simulink model "ATRIAS_vnmc"  (R2015a)
(part 22 of 23)

    (2*I^2*ddx_des*lambda1*lambda2*m*mu_s + L1^2*ddy_des*lambda2*lambda3*m^3*sin(gamma1)^2 + L1^2*g*lambda2*lambda3*m^3*sin(gamma1)^2 + 2*I^2*ddy_des*lambda1*lambda2*m*mu_s^2 + 2*I^2*g*lambda1*lambda2*m*mu_s^2 + L1^2*ddx_des*lambda1*lambda3*m^3*mu_s^3*cos(gamma1)^2 + L1^2*ddy_des*lambda2*lambda3*m^3*mu_s^2*cos(gamma1)^2 + L1^2*g*lambda2*lambda3*m^3*mu_s^2*cos(gamma1)^2 + 2*d^2*ddy_des*lambda2*lambda3*m^3*mu_s^2*cos(theta)^2 + 2*d^2*g*lambda2*lambda3*m^3*mu_s^2*cos(theta)^2 + L1^2*ddx_des*lambda1*lambda3*m^3*mu_s*sin(gamma1)^2 + I*L1*ddtheta_des*lambda2*lambda3*m^2*sin(gamma1) - I*L2*ddtheta_des*lambda2*lambda3*m^2*sin(gamma2) + 2*d^2*ddx_des*lambda1*lambda3*m^3*mu_s*sin(theta)^2 + 2*L1^2*ddy_des*lambda2*lambda3*m^3*mu_s*cos(gamma1)*sin(gamma1) + 2*L1^2*g*lambda2*lambda3*m^3*mu_s*cos(gamma1)*sin(gamma1) + I*L1*ddtheta_des*lambda2*lambda3*m^2*mu_s*cos(gamma1) + I*L2*ddtheta_des*lambda2*lambda3*m^2*mu_s*cos(gamma2) + 2*d^2*ddy_des*lambda2*lambda3*m^3*mu_s*cos(theta)*sin(theta) - 2*I*d*ddtheta_des*lambda2*lambda3*m^2*mu_s*cos(theta) + 2*d^2*g*lambda2*lambda3*m^3*mu_s*cos(theta)*sin(theta) + 2*L1^2*ddx_des*lambda1*lambda3*m^3*mu_s^2*cos(gamma1)*sin(gamma1) - I*L1*ddtheta_des*lambda1*lambda3*m^2*mu_s^3*cos(gamma1) + I*L2*ddtheta_des*lambda1*lambda3*m^2*mu_s^3*cos(gamma2) - I*L1*ddtheta_des*lambda1*lambda3*m^2*mu_s^2*sin(gamma1) - I*L2*ddtheta_des*lambda1*lambda3*m^2*mu_s^2*sin(gamma2) - L1*L2*ddy_des*lambda2*lambda3*m^3*sin(gamma1)*sin(gamma2) + 2*d^2*ddx_des*lambda1*lambda3*m^3*mu_s^2*cos(theta)*sin(theta) - L1*L2*g*lambda2*lambda3*m^3*sin(gamma1)*sin(gamma2) + 2*I*d*ddtheta_des*lambda1*lambda3*m^2*mu_s^2*sin(theta) - L1*d*ddy_des*lambda2*lambda3*m^3*sin(gamma1)*sin(theta) + L2*d*ddy_des*lambda2*lambda3*m^3*sin(gamma2)*sin(theta) - L1*d*g*lambda2*lambda3*m^3*sin(gamma1)*sin(theta) + L2*d*g*lambda2*lambda3*m^3*sin(gamma2)*sin(theta) - L1*L2*ddy_des*lambda2*lambda3*m^3*mu_s*cos(gamma1)*sin(gamma2) + L1*L2*ddy_des*lambda2*lambda3*m^3*mu_s*cos(gamma2)*sin(gamma1) - L1*L2*g*lambda2*lambda3*m^3*mu_s*cos(gamma1)*sin(gamma2) + L1*L2*g*lambda2*lambda3*m^3*mu_s*cos(gamma2)*sin(gamma1) + L1*L2*ddx_des*lambda1*lambda3*m^3*mu_s*sin(gamma1)*sin(gamma2) - L1*d*ddy_des*lambda2*lambda3*m^3*mu_s*cos(gamma1)*sin(theta) - 3*L1*d*ddy_des*lambda2*lambda3*m^3*mu_s*cos(theta)*sin(gamma1) - L2*d*ddy_des*lambda2*lambda3*m^3*mu_s*cos(gamma2)*sin(theta) + L2*d*ddy_des*lambda2*lambda3*m^3*mu_s*cos(theta)*sin(gamma2) - L1*d*g*lambda2*lambda3*m^3*mu_s*cos(gamma1)*sin(theta) - 3*L1*d*g*lambda2*lambda3*m^3*mu_s*cos(theta)*sin(gamma1) - L2*d*g*lambda2*lambda3*m^3*mu_s*cos(gamma2)*sin(theta) + L2*d*g*lambda2*lambda3*m^3*mu_s*cos(theta)*sin(gamma2) - 3*L1*d*ddx_des*lambda1*lambda3*m^3*mu_s*sin(gamma1)*sin(theta) - L2*d*ddx_des*lambda1*lambda3*m^3*mu_s*sin(gamma2)*sin(theta) - L1*L2*ddx_des*lambda1*lambda3*m^3*mu_s^3*cos(gamma1)*cos(gamma2) + L1*L2*ddy_des*lambda2*lambda3*m^3*mu_s^2*cos(gamma1)*cos(gamma2) + L1*L2*g*lambda2*lambda3*m^3*mu_s^2*cos(gamma1)*cos(gamma2) + L1*L2*ddx_des*lambda1*lambda3*m^3*mu_s^2*cos(gamma1)*sin(gamma2) - L1*L2*ddx_des*lambda1*lambda3*m^3*mu_s^2*cos(gamma2)*sin(gamma1) - L1*d*ddx_des*lambda1*lambda3*m^3*mu_s^3*cos(gamma1)*cos(theta) + L2*d*ddx_des*lambda1*lambda3*m^3*mu_s^3*cos(gamma2)*cos(theta) - 3*L1*d*ddy_des*lambda2*lambda3*m^3*mu_s^2*cos(gamma1)*cos(theta) - L2*d*ddy_des*lambda2*lambda3*m^3*mu_s^2*cos(gamma2)*cos(theta) - 3*L1*d*g*lambda2*lambda3*m^3*mu_s^2*cos(gamma1)*cos(theta) - L2*d*g*lambda2*lambda3*m^3*mu_s^2*cos(gamma2)*cos(theta) - 3*L1*d*ddx_des*lambda1*lambda3*m^3*mu_s^2*cos(gamma1)*sin(theta) - L1*d*ddx_des*lambda1*lambda3*m^3*mu_s^2*cos(theta)*sin(gamma1) + L2*d*ddx_des*lambda1*lambda3*m^3*mu_s^2*cos(gamma2)*sin(theta) - L2*d*ddx_des*lambda1*lambda3*m^3*mu_s^2*cos(theta)*sin(gamma2))/(4*I^2*lambda1*lambda2*mu_s^2 + L1^2*lambda2*lambda3*m^2*sin(gamma1)^2 + L2^2*lambda2*lambda3*m^2*sin(gamma2)^2 + L1^2*lambda2*lambda3*m^2*mu_s^2*cos(gamma1)^2 + L1^2*lambda1*lambda3*m^2*mu_s^4*cos(gamma1)^2 + L2^2*lambda2*lambda3*m^2*mu_s^2*cos(gamma2)^2 + L2^2*lambda1*lambda3*m^2*mu_s^4*cos(gamma2)^2 + L1^2*lambda1*lambda3*m^2*mu_s^2*sin(gamma1)^2 + L2^2*lambda1*lambda3*m^2*mu_s^2*sin(gamma2)^2 + 4*d^2*lambda2*lambda3*m^2*mu_s^2*cos(theta)^2 + 4*d^2*lambda1*lambda3*m^2*mu_s^2*sin(theta)^2 + 2*L1^2*lambda1*lambda3*m^2*mu_s^3*cos(gamma1)*sin(gamma1) - 2*L2^2*lambda1*lambda3*m^2*mu_s^3*cos(gamma2)*sin(gamma2) - 2*L1*L2*lambda2*lambda3*m^2*sin(gamma1)*sin(gamma2) + 2*L1^2*lambda2*lambda3*m^2*mu_s*cos(gamma1)*sin(gamma1) - 2*L2^2*lambda2*lambda3*m^2*mu_s*cos(gamma2)*sin(gamma2) + 2*L1*L2*lambda1*lambda3*m^2*mu_s^3*cos(gamma1)*sin(gamma2) - 2*L1*L2*lambda1*lambda3*m^2*mu_s^3*cos(gamma2)*sin(gamma1) + 2*L1*L2*lambda1*lambda3*m^2*mu_s^2*sin(gamma1)*sin(gamma2) - 4*L1*d*lambda2*lambda3*m^2*mu_s^2*cos(gamma1)*cos(theta) - 4*L2*d*lambda2*lambda3*m^2*mu_s^2*cos(gamma2)*cos(theta) - 4*L1*d*lambda1*lambda3*m^2*mu_s^3*cos(gamma1)*sin(theta) + 4*L2*d*lambda1*lambda3*m^2*mu_s^3*cos(gamma2)*sin(theta) - 4*L1*d*lambda1*lambda3*m^2*mu_s^2*sin(gamma1)*sin(theta) - 4*L2*d*lambda1*lambda3*m^2*mu_s^2*sin(gamma2)*sin(theta) - 2*L1*L2*lambda2*lambda3*m^2*mu_s*cos(gamma1)*sin(gamma2) + 2*L1*L2*lambda2*lambda3*m^2*mu_s*cos(gamma2)*sin(gamma1) - 4*L1*d*lambda2*lambda3*m^2*mu_s*cos(theta)*sin(gamma1) + 4*L2*d*lambda2*lambda3*m^2*mu_s*cos(theta)*sin(gamma2) + 2*L1*L2*lambda2*lambda3*m^2*mu_s^2*cos(gamma1)*cos(gamma2) - 2*L1*L2*lambda1*lambda3*m^2*mu_s^4*cos(gamma1)*cos(gamma2));
    -(2*I^2*ddx_des*lambda1*lambda2*m*mu_s - L1^2*ddy_des*lambda2*lambda3*m^3*sin(gamma1)^2 - L1^2*g*lambda2*lambda3*m^3*sin(gamma1)^2 - 2*I^2*ddy_des*lambda1*lambda2*m*mu_s^2 - 2*I^2*g*lambda1*lambda2*m*mu_s^2 + L1^2*ddx_des*lambda1*lambda3*m^3*mu_s^3*cos(gamma1)^2 - L1^2*ddy_des*lambda2*lambda3*m^3*mu_s^2*cos(gamma1)^2 - L1^2*g*lambda2*lambda3*m^3*mu_s^2*cos(gamma1)^2 - 2*d^2*ddy_des*lambda2*lambda3*m^3*mu_s^2*cos(theta)^2 - 2*d^2*g*lambda2*lambda3*m^3*mu_s^2*cos(theta)^2 + L1^2*ddx_des*lambda1*lambda3*m^3*mu_s*sin(gamma1)^2 - I*L1*ddtheta_des*lambda2*lambda3*m^2*sin(gamma1) + I*L2*ddtheta_des*lambda2*lambda3*m^2*sin(gamma2) + 2*d^2*ddx_des*lambda1*lambda3*m^3*mu_s*sin(theta)^2 + 2*L1^2*ddy_des*lambda2*lambda3*m^3*mu_s*cos(gamma1)*sin(gamma1) + 2*L1^2*g*lambda2*lambda3*m^3*mu_s*cos(gamma1)*sin(gamma1) + I*L1*ddtheta_des*lambda2*lambda3*m^2*mu_s*cos(gamma1) + I*L2*ddtheta_des*lambda2*lambda3*m^2*mu_s*cos(gamma2) + 2*d^2*ddy_des*lambda2*lambda3*m^3*mu_s*cos(theta)*sin(theta) - 2*I*d*ddtheta_des*lambda2*lambda3*m^2*mu_s*cos(theta) + 2*d^2*g*lambda2*lambda3*m^3*mu_s*cos(theta)*sin(theta) - 2*L1^2*ddx_des*lambda1*lambda3*m^3*mu_s^2*cos(gamma1)*sin(gamma1) - I*L1*ddtheta_des*lambda1*lambda3*m^2*mu_s^3*cos(gamma1) + I*L2*ddtheta_des*lambda1*lambda3*m^2*mu_s^3*cos(gamma2) + I*L1*ddtheta_des*lambda1*lambda3*m^2*mu_s^2*sin(gamma1) + I*L2*ddtheta_des*lambda1*lambda3*m^2*mu_s^2*sin(gamma2) + L1*L2*ddy_des*lambda2*lambda3*m^3*sin(gamma1)*sin(gamma2) - 2*d^2*ddx_des*lambda1*lambda3*m^3*mu_s^2*cos(theta)*sin(theta) + L1*L2*g*lambda2*lambda3*m^3*sin(gamma1)*sin(gamma2) - 2*I*d*ddtheta_des*lambda1*lambda3*m^2*mu_s^2*sin(theta) + L1*d*ddy_des*lambda2*lambda3*m^3*sin(gamma1)*sin(theta) - L2*d*ddy_des*lambda2*lambda3*m^3*sin(gamma2)*sin(theta) + L1*d*g*lambda2*lambda3*m^3*sin(gamma1)*sin(theta) - L2*d*g*lambda2*lambda3*m^3*sin(gamma2)*sin(theta) - L1*L2*ddy_des*lambda2*lambda3*m^3*mu_s*cos(gamma1)*sin(gamma2) + L1*L2*ddy_des*lambda2*lambda3*m^3*mu_s*cos(gamma2)*sin(gamma1) - L1*L2*g*lambda2*lambda3*m^3*mu_s*cos(gamma1)*sin(gamma2) + L1*L2*g*lambda2*lambda3*m^3*mu_s*cos(gamma2)*sin(gamma1) + L1*L2*ddx_des*lambda1*lambda3*m^3*mu_s*sin(gamma1)*sin(gamma2) - L1*d*ddy_des*lambda2*lambda3*m^3*mu_s*cos(gamma1)*sin(theta) - 3*L1*d*ddy_des*lambda2*lambda3*m^3*mu_s*cos(theta)*sin(gamma1) - L2*d*ddy_des*lambda2*lambda3*m^3*mu_s*cos(gamma2)*sin(theta) + L2*d*ddy_des*lambda2*lambda3*m^3*mu_s*cos(theta)*sin(gamma2) - L1*d*g*lambda2*lambda3*m^3*mu_s*cos(gamma1)*sin(theta) - 3*L1*d*g*lambda2*lambda3*m^3*mu_s*cos(theta)*sin(gamma1) - L2*d*g*lambda2*lambda3*m^3*mu_s*cos(gamma2)*sin(theta) + L2*d*g*lambda2*lambda3*m^3*mu_s*cos(theta)*sin(gamma2) - 3*L1*d*ddx_des*lambda1*lambda3*m^3*mu_s*sin(gamma1)*sin(theta) - L2*d*ddx_des*lambda1*lambda3*m^3*mu_s*sin(gamma2)*sin(theta) - L1*L2*ddx_des*lambda1*lambda3*m^3*mu_s^3*cos(gamma1)*cos(gamma2) - L1*L2*ddy_des*lambda2*lambda3*m^3*mu_s^2*cos(gamma1)*cos(gamma2) - L1*L2*g*lambda2*lambda3*m^3*mu_s^2*cos(gamma1)*cos(gamma2) - L1*L2*ddx_des*lambda1*lambda3*m^3*mu_s^2*cos(gamma1)*sin(gamma2) + L1*L2*ddx_des*lambda1*lambda3*m^3*mu_s^2*cos(gamma2)*sin(gamma1) - L1*d*ddx_des*lambda1*lambda3*m^3*mu_s^3*cos(gamma1)*cos(theta) + L2*d*ddx_des*lambda1*lambda3*m^3*mu_s^3*cos(gamma2)*cos(theta) + 3*L1*d*ddy_des*lambda2*lambda3*m^3*mu_s^2*cos(gamma1)*cos(theta) + L2*d*ddy_des*lambda2*lambda3*m^3*mu_s^2*cos(gamma2)*cos(theta) + 3*L1*d*g*lambda2*lambda3*m^3*mu_s^2*cos(gamma1)*cos(theta) + L2*d*g*lambda2*lambda3*m^3*mu_s^2*cos(gamma2)*cos(theta) + 3*L1*d*ddx_des*lambda1*lambda3*m^3*mu_s^2*cos(gamma1)*sin(theta) + L1*d*ddx_des*lambda1*lambda3*m^3*mu_s^2*cos(theta)*sin(gamma1) - L2*d*ddx_des*lambda1*lambda3*m^3*mu_s^2*cos(gamma2)*sin(theta) + L2*d*ddx_des*lambda1*lambda3*m^3*mu_s^2*cos(theta)*sin(gamma2))/(4*I^2*lambda1*lambda2*mu_s^2 + L1^2*lambda2*lambda3*m^2*sin(gamma1)^2 + L2^2*lambda2*lambda3*m^2*sin(gamma2)^2 + L1^2*lambda2*lambda3*m^2*mu_s^2*cos(gamma1)^2 + L1^2*lambda1*lambda3*m^2*mu_s^4*cos(gamma1)^2 + L2^2*lambda2*lambda3*m^2*mu_s^2*cos(gamma2)^2 + L2^2*lambda1*lambda3*m^2*mu_s^4*cos(gamma2)^2 + L1^2*lambda1*lambda3*m^2*mu_s^2*sin(gamma1)^2 + L2^2*lambda1*lambda3*m^2*mu_s^2*sin(gamma2)^2 + 4*d^2*lambda2*lambda3*m^2*mu_s^2*cos(theta)^2 + 4*d^2*lambda1*lambda3*m^2*mu_s^2*sin(theta)^2 - 2*L1^2*lambda1*lambda3*m^2*mu_s^3*cos(gamma1)*sin(gamma1) + 2*L2^2*lambda1*lambda3*m^2*mu_s^3*cos(gamma2)*sin(gamma2) - 2*L1*L2*lambda2*lambda3*m^2*sin(gamma1)*sin(gamma2) - 2*L1^2*lambda2*lambda3*m^2*mu_s*cos(gamma1)*sin(gamma1) + 2*L2^2*lambda2*lambda3*m^2*mu_s*cos(gamma2)*sin(gamma2) - 2*L1*L2*lambda1*lambda3*m^2*mu_s^3*cos(gamma1)*sin(gamma2) + 2*L1*L2*lambda1*lambda3*m^2*mu_s^3*cos(gamma2)*sin(gamma1) + 2*L1*L2*lambda1*lambda3*m^2*mu_s^2*sin(gamma1)*sin(gamma2) - 4*L1*d*lambda2*lambda3*m^2*mu_s^2*cos(gamma1)*cos(theta) - 4*L2*d*lambda2*lambda3*m^2*mu_s^2*cos(gamma2)*cos(theta) + 4*L1*d*lambda1*lambda3*m^2*mu_s^3*cos(gamma1)*sin(theta) - 4*L2*d*lambda1*lambda3*m^2*mu_s^3*cos(gamma2)*sin(theta) - 4*L1*d*lambda1*lambda3*m^2*mu_s^2*sin(gamma1)*sin(theta) - 4*L2*d*lambda1*lambda3*m^2*mu_s^2*sin(gamma2)*sin(theta) + 2*L1*L2*lambda2*lambda3*m^2*mu_s*cos(gamma1)*sin(gamma2) - 2*L1*L2*lambda2*lambda3*m^2*mu_s*cos(gamma2)*sin(gamma1) + 4*L1*d*lambda2*lambda3*m^2*mu_s*cos(theta)*sin(gamma1) - 4*L2*d*lambda2*lambda3*m^2*mu_s*cos(theta)*sin(gamma2) + 2*L1*L2*lambda2*lambda3*m^2*mu_s^2*cos(gamma1)*cos(gamma2) - 2*L1*L2*lambda1*lambda3*m^2*mu_s^4*cos(gamma1)*cos(gamma2))]);

% f1 = 0; f2 = 0; f3 = 0; f4 = 0;

% numerical precision factor 
thr = 100*eps; % (without this, solution can give suboptimal/unexpected results)

c1 = mu_s*f2-f1 >= -thr;
c2 = mu_s*f2+f1 >= -thr;
c3 = mu_s*f4-f3 >= -thr;
c4 = mu_s*f4+f3 >= -thr;
c5 = f2 >= -thr;
c6 = f4 >= -thr;

constraints = c1 & c2 & c3 & c4 & c5 & c6;
satisfied = find(constraints);

ddx = 1/m*(f1+f3);
ddy = 1/m*(f2+f4-m*g);
ddtheta = 1/I*(f1*(-d*cos(theta)+L1*cos(gamma1))+f2*(d*sin(theta)-L1*sin(gamma1))+...
    f3*(-d*cos(theta)+L2*cos(gamma2))+f4*(d*sin(theta)-L2*sin(gamma2)));

fR_mag = sqrt(f1.^2 + f2.^2);
fL_mag = sqrt(f3.^2 + f4.^2);

% F1 = lambda1*(ddx-ddx_des).^2+lambda2*(ddy-ddy_des).^2+lambda3*(ddtheta-ddtheta_des).^2;
% F1 = lambda1*(ddx-ddx_des).^2+lambda2*(ddy-ddy_des).^2+lambda3*(ddtheta-ddtheta_des).^2 + ...
%     lambda4*(abs(f1-grf_prev(1)) + abs(f2-grf_prev(2)) + abs(f3-grf_prev(3)) + abs(f4-grf_prev(4)));
% F1 = lambda1*(ddx-ddx_des).^2+lambda2*(ddy-ddy_des).^2+lambda3*(ddtheta-ddtheta_des).^2 + ...
%     lambda4*(abs(f1-grf_meas(1)) + abs(f2-grf_meas(2)) + abs(f3-grf_meas(3)) + abs(f4-grf_meas(4)));

% fR_mag_meas = sqrt(grf_meas(1)^2 + grf_meas(2)^2);
% fL_mag_meas = sqrt(grf_meas(3)^2 + grf_meas(4)^2);

F1 = lambda1*(ddx-ddx_des).^2+lambda2*(ddy-ddy_des).^2+lambda3*(ddtheta-ddtheta_des).^2 + ...
    lambda4*abs(fR_mag-fL_mag);
% F1 = lambda1*(ddx-ddx_des).^2+lambda2*(ddy-ddy_des).^2+lambda3*(ddtheta-ddtheta_des).^2 + ...
%     lambda4*(abs(fR_mag-fR_mag_meas) + abs(fL_mag-fL_mag_meas));
% 
% F1 = lambda1*(ddx-ddx_des).^2+lambda2*(ddy-ddy_des).^2+lambda3*(ddtheta-ddtheta_des).^2 + ...
%     lambda4*(abs(f1-grf_meas(1)) + abs(f2-grf_meas(2)) + abs(f3-grf_meas(3)) + abs(f4-grf_meas(4)));



% F2 = (f1-grf_prev(1)).^2 + (f2-grf_prev(2)).^2 + (f3-grf_prev(3)).^2 + (f4-grf_prev(4)).^2;
% F2 = abs(f1-grf_prev(1)) + abs(f2-grf_prev(2)) + abs(f3-grf_prev(3)) + abs(f4-grf_prev(4)) + ...
%      lambda4*((sign(f1)~= grf_prev(1))+(sign(f2)~= grf_prev(2))+...
%      (sign(f3)~= grf_prev(3))+(sign(f4)~= grf_prev(4)));
% F2 = (sign(f1)~= sign(grf_prev(1)))+(sign(f2)~= sign(grf_prev(2)))+...
%      (sign(f3)~= sign(grf_prev(3)))+(sign(f4)~= sign(grf_prev(4)));

F2 = abs(fR_mag-fL_mag);


% F1 = F1(constraints);
% F2 = F2(constraints);



% if length(F1)>1
%     [F1_sorted,F1_sorted_idx] = sort(F1);
%     diff_F1_sorted = diff(F1_sorted);
%     same_cost_idx = find(diff_F1_sorted,1);
%     
%     if isempty(same_cost_idx)
%         same_cost_idx = length(F1_sorted_idx);
%     end
%     
%     [cost,min_idx] = min(F2(F1_sorted_idx(1:same_cost_idx(1))));
%     min_idx = F1_sorted_idx(min_idx);
% else
%     [cost,min_idx] = min(F1);
% end

[M,~] = min(F1(satisfied));
if ~isempty(M)
    I = satisfied(F1(satisfied)-M <= thr);
    [cost_tie_break, I2] = min(F2(I));
    
    
%     ddx_satisfied = ddx(constraints);
%     ddy_satisfied = ddy(constraints);
%     ddtheta_satisfied = ddtheta(constraints);
    
    e_ddx = [ddx(I(I2)) - ddx_des];
    e_ddy = [ddy(I(I2)) - ddy_des];
    e_ddtheta = [ddtheta(I(I2)) - ddtheta_des];
%     e_ddx = [ddx_satisfied(min_idx) - ddx_des];
%     e_ddy = [ddy_satisfied(min_idx) - ddy_des];
%     e_ddtheta = [ddtheta_satisfied(min_idx) - ddtheta_des];
    
    err = [e_ddx e_ddy e_ddtheta];
    
    f1 = f1(I(I2));
    f2 = f2(I(I2));
    f3 = f3(I(I2));
    f4 = f4(I(I2));
%     f1 = f1(constraints); f1 = f1(min_idx);
%     f2 = f2(constraints); f2 = f2(min_idx);
%     f3 = f3(constraints); f3 = f3(min_idx);
%     f4 = f4(constraints); f4 = f4(min_idx);
    
    
    f2 = max(f2,min_Fy);
    f4 = max(f4,min_Fy);
    grf = [f1; f2; f3; f4];
        
    leg_force_hip_torque = J1*grf;
    motor_trq = J2*leg_force_hip_torque;
else
    grf = [0;0;0;0];
    err = [-ddx_des -ddy_des -ddtheta_des];
    leg_force_hip_torque = [0;0;0;0];
    motor_trq = [0;0;0;0];
end

end
